simulink model "TrabalhoReatorCaCbwal"  (R2024a)
settings: Solver=VariableStepAuto  StartTime=0.0  StopTime=40  RelTol=1e-3
values from neighbouring files (symbols this model uses):
  k1 = 6.01    [Trabalho_SC_Reator.m]
  k2 = 0.8433    [Trabalho_SC_Reator.m]
  k3 = 0.1123    [Trabalho_SC_Reator.m]
settings Model: Creator=walla  LastModifiedBy=walla

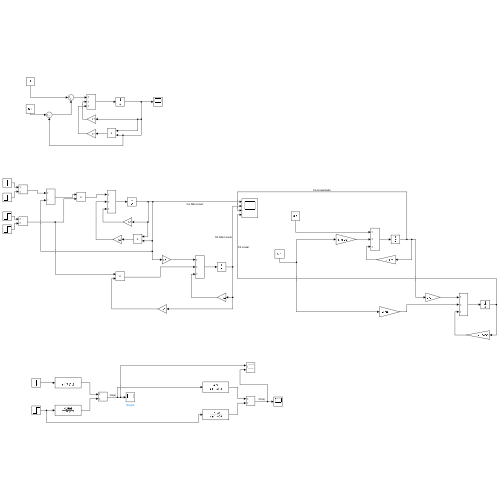
[thumbnail: Simulink's stored preview of the top-level diagram]
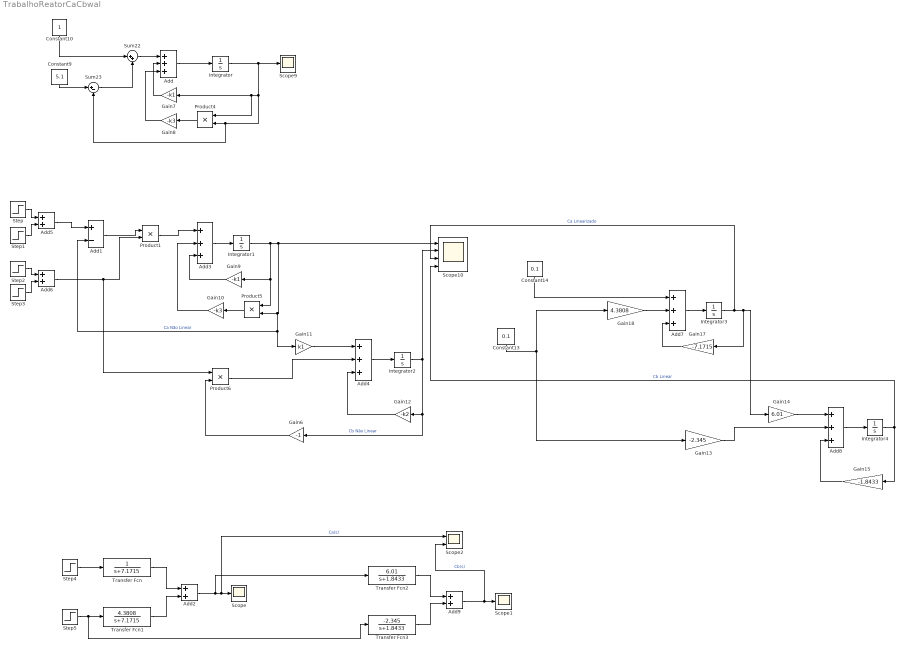
== system TrabalhoReatorCaCbwal ==
  Add{,3..4,7..8} (5 alike) : Sum  Inputs=+++
  Add1 : Sum  Inputs=+-
  Add{2,5..6,9} (4 alike) : Sum
  Constant10 : Constant
  Constant13 : Constant  Value=0.1
  Constant14 : Constant  Value=0.1
  Constant9 : Constant  Value=5.1
  Gain10 : Gain  Gain=-k3
  Gain11 : Gain  Gain=k1
  Gain12 : Gain  Gain=-k2
  Gain13 : Gain  Gain=-2.345
  Gain14 : Gain  Gain=6.01
  Gain15 : Gain  Gain=-1.8433
  Gain17 : Gain  Gain=-7.1715
  Gain18 : Gain  Gain=4.3808
  Gain6 : Gain  Gain=-1
  Gain7 : Gain  Gain=-k1
  Gain8 : Gain  Gain=-k3
  Gain9 : Gain  Gain=-k1
  Integrator{,1..4} (5 alike) : Integrator
  Product{1,4..6} (4 alike) : Product
  Scope : Scope
  Scope1 : Scope
  Scope10 : Scope  NumInputPorts=4
  Scope2 : Scope  NumInputPorts=2
  Scope9 : Scope
  Step : Step  Time=0  After=5.1  SampleTime=0
  Step1 : Step  Time=10  After=0.1  SampleTime=0
  Step2 : Step  Time=0  SampleTime=0
  Step3 : Step  Time=10  After=0.1  SampleTime=0
  Step4 : Step  Time=0  After=0.1  SampleTime=0
  Step5 : Step  Time=0  After=0.1  SampleTime=0
  Sum22 : Sum  Inputs=|++
  Sum23 : Sum  Inputs=|+-
  Transfer Fcn : TransferFcn  Denominator=[1 7.1715]
  Transfer Fcn1 : TransferFcn  Numerator=[4.3808]  Denominator=[1 7.1715]
  Transfer Fcn2 : TransferFcn  Numerator=[6.01]  Denominator=[1 1.8433]
  Transfer Fcn3 : TransferFcn  Numerator=[-2.345]  Denominator=[1 1.8433]
  wires:
  Sum23/1 -> Sum22/2
  Sum22/1 -> Add/1
  Add4/1 -> Integrator2/1
  Integrator2/1 -> Scope10/2, Gain6/1, Gain12/1  "Cb Não Linear"
  Gain9/1 -> Add3/3
  Gain11/1 -> Add4/1
  Integrator/1 -> Sum23/2, Product4/2, Product4/1, Gain7/1, Scope9/1
  Integrator1/1 -> Gain11/1, Add1/2, Product5/2, Scope10/1, Product5/1, Gain9/1  "Ca Não Linear"
  Product6/1 -> Add4/2
  Constant9/1 -> Sum23/1
  Gain10/1 -> Add3/2
  Add3/1 -> Integrator1/1
  Product4/1 -> Gain8/1
  Gain8/1 -> Add/3
  Constant10/1 -> Sum22/1
  Gain12/1 -> Add4/3
  Add/1 -> Integrator/1
  Gain7/1 -> Add/2
  Product1/1 -> Add3/1
  Product5/1 -> Gain10/1
  Gain6/1 -> Product6/2
  Constant13/1 -> Gain13/1, Gain18/1
  Gain17/1 -> Add7/3
  Gain15/1 -> Add8/3
  Add7/1 -> Integrator3/1
  Gain13/1 -> Add8/2
  Integrator3/1 -> Gain14/1, Gain17/1, Scope10/3  "Ca Linearizado"
  Integrator4/1 -> Scope10/4, Gain15/1  "Cb Linear"
  Gain14/1 -> Add8/1
  Add8/1 -> Integrator4/1
  Gain18/1 -> Add7/2
  Add1/1 -> Product1/1
  Constant14/1 -> Add7/1
  Step/1 -> Add5/1
  Step1/1 -> Add5/2
  Add5/1 -> Add1/1
  Step2/1 -> Add6/1
  Step3/1 -> Add6/2
  Add6/1 -> Product6/1, Product1/2
  Step5/1 -> Transfer Fcn3/1, Transfer Fcn1/1
  Step4/1 -> Transfer Fcn/1
  Transfer Fcn/1 -> Add2/1
  Transfer Fcn1/1 -> Add2/2
  Add2/1 -> Transfer Fcn2/1, Scope2/1, Scope/1  "Ca(s)"
  Transfer Fcn3/1 -> Add9/2
  Transfer Fcn2/1 -> Add9/1
  Add9/1 -> Scope2/2, Scope1/1  "Cb(s)"
